simulink library "Input_Water"  (Simulink 8.2)
settings: Solver=ode45  StartTime=0.0  StopTime=10.0  RelTol=1e-3
settings Model: Creator=lena.frank  LastModifiedBy=drhf

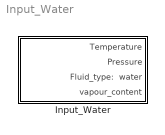
== system Input_Water ==
  Input_Water : Subsystem  mask(Input_Water){T=20, p=2e6, xd=0}
      mask prompts: T "temperature (scalar or vector) [°C]"; p "pressure [Pa]"; xd "vapour content of the water [0..1]"
      mask help:
      | Input block for the material "Water"
      |
      | The relevant inputs for the calculation of the block can be specified as parameter in the mask
      mask Help: web(fullfile(path_carnot('help'),'input_material.html'),'-helpbrowser')

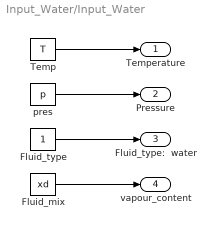
== system Input_Water/Input_Water ==
  Fluid_mix : Constant  Value=xd
  Fluid_type : Constant
  Temp : Constant  Value=T
  pres : Constant  Value=p
  Temperature : Outport
  Pressure : Outport  Port=2
  Fluid_type:  water : Outport  Port=3
  vapour_content : Outport  Port=4
  wires:
  Fluid_mix/1 -> vapour_content/1
  Fluid_type/1 -> Fluid_type:  water/1
  Temp/1 -> Temperature/1
  pres/1 -> Pressure/1
